simulink model "mytopologybat"  (R2014b)
settings: Solver=ode23tb  StartTime=0.0  StopTime=1  MaxStep=0.0001  MinStep=0.00001  RelTol=1e-3
libraries: powerlib x130, simulink x45, powerlib_meascontrol x2
(part 1 of 2)
settings Model: Creator=HOME  LastModifiedBy=SELVA
settings DataIOCC: SignalLoggingSaveFormat=ModelDataLogs
settings OptimizationCC: ExpressionDepthLimit=2147483647
settings DebuggingCC: UnderspecifiedInitializationDetection=Classic  MergeDetectMultiDrivingBlocksExec=none  FcnCallInpInsideContextMsg=UseLocalSettings  StateNameClashWarn=warning
settings GRTTargetCC: CombineOutputUpdateFcns=off  GRTInterface=on

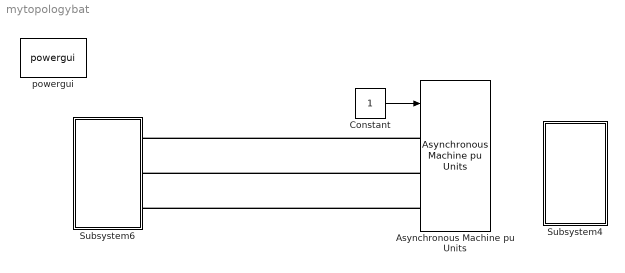
== system mytopologybat ==
  Asynchronous Machine pu Units : powerlib/Machines/Asynchronous Machine pu Units  PresetModel=No  MechanicalLoad=Torque Tm  ShowDetailedParameters=on  RotorType=Squirrel-cage  ReferenceFrame=Rotor  Units=pu  MeasurementBus=off  NominalParameters=[3730 460 60]  Stator=[0.01965 0.0397]  Rotor=[0.01909 0.0397]  Cage1=[0.01909 0.0397]  Cage2=[0.01909 0.0397]  Lm=1.354  Mechanical=[0.09526 0.05479 2]  PolePairs=2  InitialConditions="[ 1,0   0,0,0   0,0,0 ]"  SimulateSaturation=off  Saturation="[0.212,0.4201,0.8125,1.0979,1.4799,2.2457,3.2586,4.5763,6.4763 ;   0.5,0.7,0.9,1,1.1,1.2 ,1.3,1.4,1.5]"  LoadFlowParameters=0  TsPowergui=0  TsBlock=-1  IterativeModel=Trapezoidal non iterative  Pmec=0
  Constant : Constant
  Subsystem4 : Subsystem
  Subsystem6 : Subsystem  mask{m=1, fc=1000, v=230, c1=48}
      mask prompts: m "Modulation Index"; fc "Switching Frequency"; v "1 Phase Input Voltage"; c1 "DC Link Capacitor"
  powergui : powerlib/powergui  Priority=1  SimulationMode=Discrete  SolverType=Tustin/Backward Euler (TBE)  SampleTime=50e-6  frequency=60  SPID=off  DisableSnubberDevices=off  DisableRonSwitches=off  DisableVfSwitches=off  SwTol=0  DisplayEquations=off  Interpol=off  methode=off  Ts=100  frequencyindice=0  Pbase=100e6  ErrMax=1e-4  Iterations=50  UnitsV=kV  UnitsW=MW  FunctionMessages=off  echomessages=off  HookPort=off  EnableUseOfTLC=off  x0status=blocks  RestoreLinks=warning  ResistiveCurrentMeasurement=off  Frange=[0:2:500]  Ylog=off  Xlog=on  ShowGrid=off  save=off  variable=ZData  structure=ScopeData1  ZoomFFT=off  StartTime=0.1  cycles=1  DisplayStyle=1  fundamental=50  FreqAxis=off  MaxFrequency=1000  frequencyindicesteady=1  RmsSteady=1  display=off
  wires:
  Constant/1 -> Asynchronous Machine pu Units/1
  connections:
  Asynchronous Machine pu Units/LConn1 -- Subsystem6/RConn1
  Asynchronous Machine pu Units/LConn2 -- Subsystem6/RConn2
  Asynchronous Machine pu Units/LConn3 -- Subsystem6/RConn3

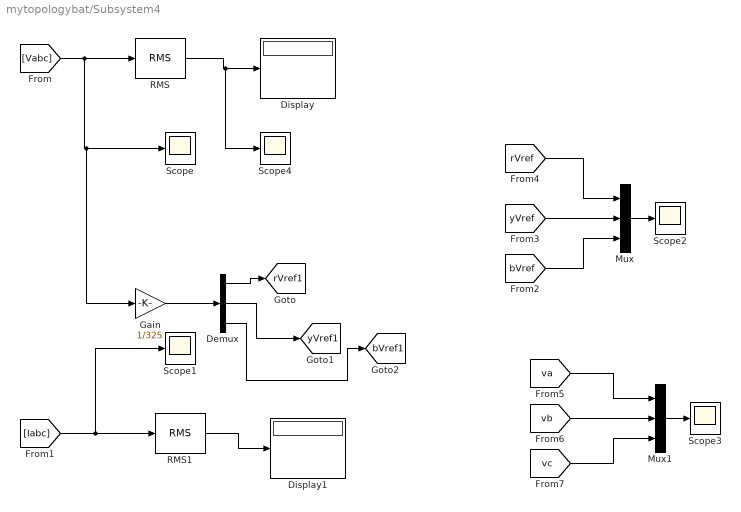
== system mytopologybat/Subsystem4 ==
  Demux : Demux  Outputs=3
  Display : Display
  Display1 : Display
  Gain : Gain  Gain=1/325
  Mux : Mux  Inputs=3
  Mux1 : Mux  Inputs=3
  RMS : powerlib_meascontrol/Measurements/RMS  TrueRMS=on  Freq=50  RMSInit=120  Ts=0
  RMS1 : powerlib_meascontrol/Measurements/RMS  TrueRMS=on  Freq=50  RMSInit=120  Ts=0
  Scope{,1..4} (5 alike) : Scope
      Scope settings: YMin=-400  YMax=400
      Scope1 settings: YMin=-600  YMax=800  SaveName=ScopeData2
      Scope2 settings: YMin=-8  YMax=8  SaveName=ScopeData4
      Scope3 settings: YMin=-400  YMax=400
      Scope4 settings: YMin=-600  YMax=600  SaveName=ScopeData3
  tag scope: bVref1=global, rVref1=global, yVref1=global
  wires:
  [Vabc] -> Gain/1, Scope/1, RMS/1
  RMS/1 -> Scope4/1, Display/1
  RMS1/1 -> Display1/1
  Mux/1 -> Scope2/1
  [bVref] -> Mux/3
  [rVref] -> Mux/1
  [yVref] -> Mux/2
  Mux1/1 -> Scope3/1
  [vc] -> Mux1/3
  [vb] -> Mux1/2
  [va] -> Mux1/1
  [Iabc] -> RMS1/1, Scope1/1
  Demux/1 -> [rVref1]
  Demux/2 -> [yVref1]
  Demux/3 -> [bVref1]
  Gain/1 -> Demux/1

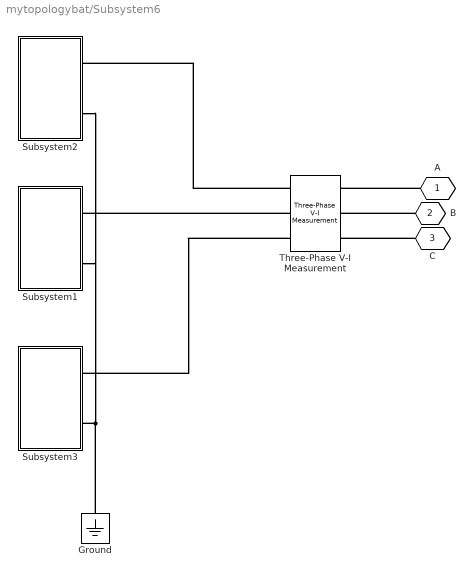
== system mytopologybat/Subsystem6 ==
  Ground : powerlib/Elements/Ground  LConnTagsString=a
  Subsystem1 : Subsystem
  Subsystem2 : Subsystem
  Subsystem3 : Subsystem
  Three-Phase V-I Measurement : powerlib/Measurements/Three-Phase V-I Measurement  VoltageMeasurement=phase-to-ground  SetLabelV=on  LabelV=Vabc  Vpu=off  VpuLL=off  CurrentMeasurement=yes  SetLabelI=on  LabelI=Iabc  Ipu=off  Pbase=100e6  Vbase=500e3  OutputType=Complex  PhasorSimulation=off  PSBequivalent=0
  A : PMIOPort  Port=1  Side=Right
  B : PMIOPort  Port=2  Side=Right
  C : PMIOPort  Port=3  Side=Right
  connections:
  Subsystem3/RConn2 -- Ground/LConn1 -- Subsystem2/RConn2 -- Subsystem1/RConn2
  Three-Phase V-I Measurement/LConn3 -- Subsystem3/RConn1
  Three-Phase V-I Measurement/LConn2 -- Subsystem1/RConn1
  Three-Phase V-I Measurement/LConn1 -- Subsystem2/RConn1
  A/RConn1 -- Three-Phase V-I Measurement/RConn1
  B/RConn1 -- Three-Phase V-I Measurement/RConn2
  C/RConn1 -- Three-Phase V-I Measurement/RConn3

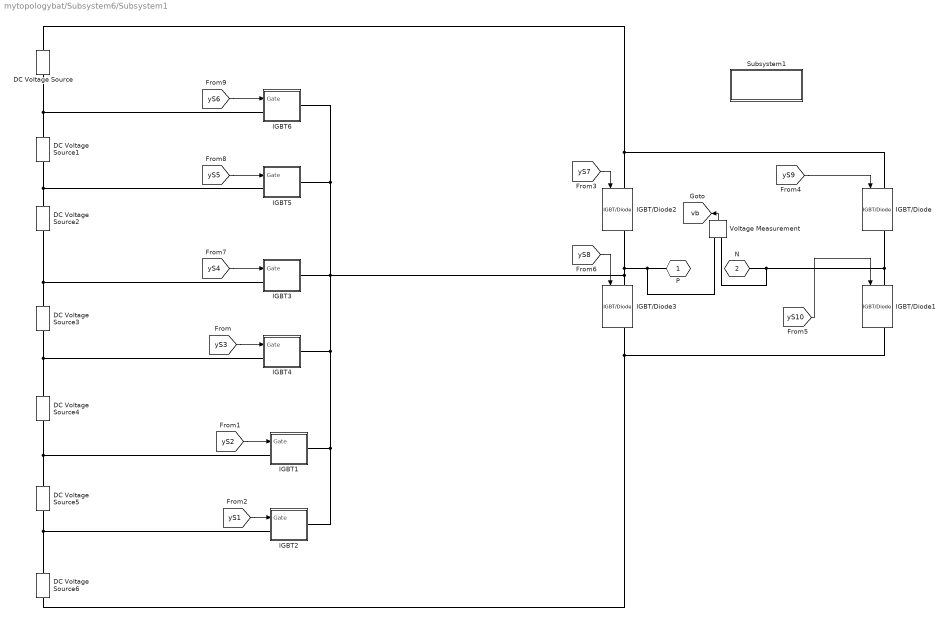
== system mytopologybat/Subsystem6/Subsystem1 ==
  DC Voltage Source{,1..6} (7 alike) : powerlib/Electrical Sources/DC Voltage Source  Amplitude=c1  Measurements=None
  IGBT/Diode{,1..3} (4 alike) : powerlib/Power Electronics/IGBT//Diode  Ron=1e-3  Rs=1e5  Cs=inf  Measurements=on
  IGBT1 : Subsystem
  IGBT2 : Subsystem
  IGBT3 : Subsystem
  IGBT4 : Subsystem
  IGBT5 : Subsystem
  IGBT6 : Subsystem
  Subsystem1 : Subsystem
  Voltage Measurement : powerlib/Measurements/Voltage Measurement  PhasorSimulation=off  OutputType=Complex  PSBequivalent=0
  P : PMIOPort  Port=1  Side=Right
  N : PMIOPort  Port=2  Side=Right
  tag scope: vb=global
  wires:
  [yS8] -> IGBT/Diode3/1
  [yS7] -> IGBT/Diode2/1
  [yS10] -> IGBT/Diode1/1
  [yS9] -> IGBT/Diode/1
  [yS1] -> IGBT2/1(Gate)
  [yS3] -> IGBT4/1(Gate)
  [yS2] -> IGBT1/1(Gate)
  [yS4] -> IGBT3/1(Gate)
  [yS5] -> IGBT5/1(Gate)
  [yS6] -> IGBT6/1(Gate)
  Voltage Measurement/1 -> [vb]
  connections:
  N/RConn1 -- IGBT/Diode/RConn1 -- IGBT/Diode1/LConn1 -- Voltage Measurement/LConn2
  IGBT/Diode3/RConn1 -- IGBT/Diode1/RConn1 -- DC Voltage Source6/LConn1
  IGBT2/RConn1 -- IGBT/Diode3/LConn1 -- Voltage Measurement/LConn1 -- P/RConn1 -- IGBT/Diode2/RConn1 -- IGBT6/RConn1 -- IGBT5/RConn1 -- IGBT3/RConn1 -- IGBT4/RConn1 -- IGBT1/RConn1
  IGBT/Diode2/LConn1 -- DC Voltage Source/RConn1 -- IGBT/Diode/LConn1
  DC Voltage Source4/RConn1 -- DC Voltage Source3/LConn1 -- IGBT4/LConn1
  DC Voltage Source5/RConn1 -- IGBT1/LConn1 -- DC Voltage Source4/LConn1
  DC Voltage Source5/LConn1 -- IGBT2/LConn1 -- DC Voltage Source6/RConn1
  DC Voltage Source/LConn1 -- IGBT6/LConn1 -- DC Voltage Source1/RConn1
  DC Voltage Source3/RConn1 -- DC Voltage Source2/LConn1 -- IGBT3/LConn1
  DC Voltage Source2/RConn1 -- DC Voltage Source1/LConn1 -- IGBT5/LConn1

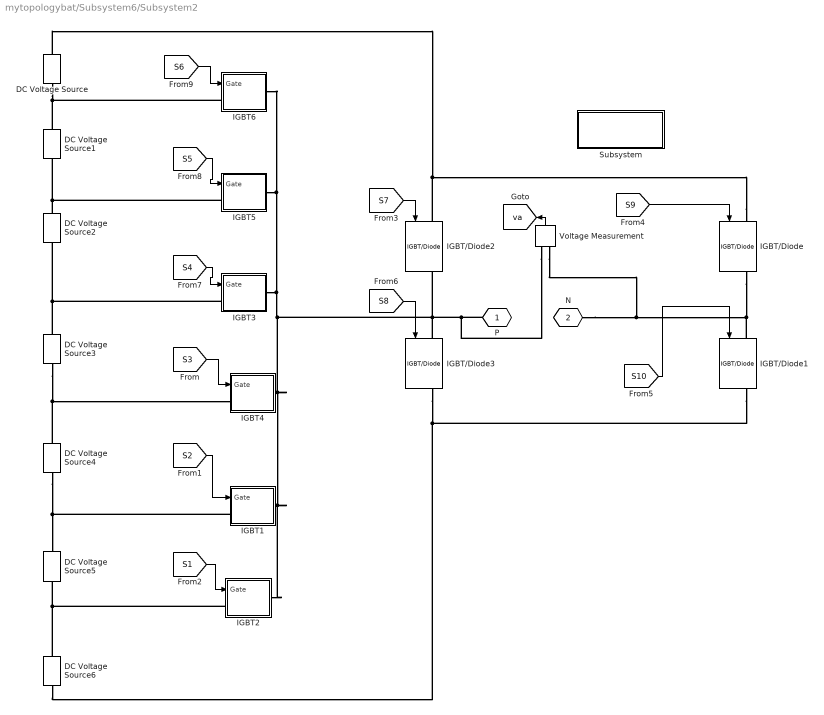
== system mytopologybat/Subsystem6/Subsystem2 ==
  DC Voltage Source{,1..6} (7 alike) : powerlib/Electrical Sources/DC Voltage Source  Amplitude=c1  Measurements=None
  IGBT/Diode{,1..3} (4 alike) : powerlib/Power Electronics/IGBT//Diode  Ron=1e-3  Rs=1e5  Cs=inf  Measurements=on
  IGBT1 : Subsystem
  IGBT2 : Subsystem
  IGBT3 : Subsystem
  IGBT4 : Subsystem
  IGBT5 : Subsystem
  IGBT6 : Subsystem
  Subsystem : Subsystem
  Voltage Measurement : powerlib/Measurements/Voltage Measurement  PhasorSimulation=off  OutputType=Complex  PSBequivalent=0
  P : PMIOPort  Port=1  Side=Right
  N : PMIOPort  Port=2  Side=Right
  tag scope: va=global
  wires:
  [S2] -> IGBT1/1(Gate)
  [S3] -> IGBT4/1(Gate)
  [S1] -> IGBT2/1(Gate)
  [S9] -> IGBT/Diode/1
  [S10] -> IGBT/Diode1/1
  [S7] -> IGBT/Diode2/1
  [S8] -> IGBT/Diode3/1
  [S4] -> IGBT3/1(Gate)
  [S5] -> IGBT5/1(Gate)
  [S6] -> IGBT6/1(Gate)
  Voltage Measurement/1 -> [va]
  connections:
  DC Voltage Source4/RConn1 -- DC Voltage Source3/LConn1 -- IGBT4/LConn1
  IGBT1/LConn1 -- DC Voltage Source4/LConn1 -- DC Voltage Source5/RConn1
  IGBT/Diode/LConn1 -- DC Voltage Source/RConn1 -- IGBT/Diode2/LConn1
  IGBT/Diode3/LConn1 -- Voltage Measurement/LConn1 -- P/RConn1 -- IGBT4/RConn1 -- IGBT2/RConn1 -- IGBT1/RConn1 -- IGBT6/RConn1 -- IGBT5/RConn1 -- IGBT3/RConn1 -- IGBT/Diode2/RConn1
  IGBT2/LConn1 -- DC Voltage Source6/RConn1 -- DC Voltage Source5/LConn1
  IGBT/Diode1/RConn1 -- DC Voltage Source6/LConn1 -- IGBT/Diode3/RConn1
  IGBT/Diode/RConn1 -- Voltage Measurement/LConn2 -- N/RConn1 -- IGBT/Diode1/LConn1
  IGBT6/LConn1 -- DC Voltage Source1/RConn1 -- DC Voltage Source/LConn1
  IGBT3/LConn1 -- DC Voltage Source3/RConn1 -- DC Voltage Source2/LConn1
  DC Voltage Source2/RConn1 -- DC Voltage Source1/LConn1 -- IGBT5/LConn1

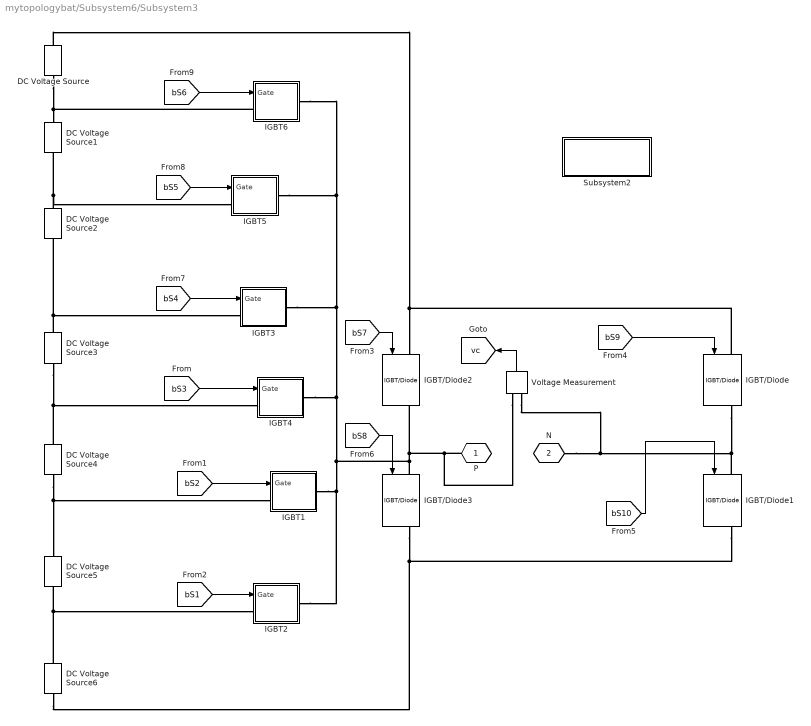
== system mytopologybat/Subsystem6/Subsystem3 ==
  DC Voltage Source{,1..6} (7 alike) : powerlib/Electrical Sources/DC Voltage Source  Amplitude=c1  Measurements=None
  IGBT/Diode{,1..3} (4 alike) : powerlib/Power Electronics/IGBT//Diode  Ron=1e-3  Rs=1e5  Cs=inf  Measurements=on
  IGBT1 : Subsystem
  IGBT2 : Subsystem
  IGBT3 : Subsystem
  IGBT4 : Subsystem
  IGBT5 : Subsystem
  IGBT6 : Subsystem
  Subsystem2 : Subsystem
  Voltage Measurement : powerlib/Measurements/Voltage Measurement  PhasorSimulation=off  OutputType=Complex  PSBequivalent=0
  P : PMIOPort  Port=1  Side=Right
  N : PMIOPort  Port=2  Side=Right
  tag scope: vc=global
  wires:
  [bS2] -> IGBT1/1(Gate)
  [bS3] -> IGBT4/1(Gate)
  [bS1] -> IGBT2/1(Gate)
  [bS9] -> IGBT/Diode/1
  [bS10] -> IGBT/Diode1/1
  [bS7] -> IGBT/Diode2/1
  [bS8] -> IGBT/Diode3/1
  [bS4] -> IGBT3/1(Gate)
  [bS5] -> IGBT5/1(Gate)
  [bS6] -> IGBT6/1(Gate)
  Voltage Measurement/1 -> [vc]
  connections:
  IGBT/Diode/LConn1 -- DC Voltage Source/RConn1 -- IGBT/Diode2/LConn1
  P/RConn1 -- Voltage Measurement/LConn1 -- IGBT/Diode2/RConn1 -- IGBT/Diode3/LConn1 -- IGBT6/RConn1 -- IGBT5/RConn1 -- IGBT3/RConn1 -- IGBT4/RConn1 -- IGBT1/RConn1 -- IGBT2/RConn1
  IGBT/Diode3/RConn1 -- DC Voltage Source6/LConn1 -- IGBT/Diode1/RConn1
  IGBT/Diode1/LConn1 -- Voltage Measurement/LConn2 -- N/RConn1 -- IGBT/Diode/RConn1
  DC Voltage Source4/RConn1 -- DC Voltage Source3/LConn1 -- IGBT4/LConn1
  DC Voltage Source4/LConn1 -- DC Voltage Source5/RConn1 -- IGBT1/LConn1
  DC Voltage Source5/LConn1 -- IGBT2/LConn1 -- DC Voltage Source6/RConn1
  DC Voltage Source/LConn1 -- IGBT6/LConn1 -- DC Voltage Source1/RConn1
  DC Voltage Source3/RConn1 -- DC Voltage Source2/LConn1 -- IGBT3/LConn1
  DC Voltage Source2/RConn1 -- IGBT5/LConn1 -- DC Voltage Source1/LConn1

== system mytopologybat/Subsystem6/Subsystem1/IGBT1 ==
  Gate : Inport
  Diode{,1..3} (4 alike) : powerlib/Power Electronics/Diode  Ron=0.001  Lon=0  Vf=0.8  IC=0  UseSnubber=off  Rs=500  Cs=250e-9  Measurements=on
  IGBT/Diode : powerlib/Power Electronics/IGBT//Diode  Ron=1e-3  Rs=1e5  Cs=inf  Measurements=on
  C : PMIOPort  Port=1  Side=Left
  E : PMIOPort  Port=2  Side=Right
  wires:
  Gate/1 -> IGBT/Diode/1
  connections:
  Diode/RConn1 -- Diode2/RConn1 -- IGBT/Diode/LConn1
  Diode1/LConn1 -- Diode3/LConn1 -- IGBT/Diode/RConn1
  Diode2/LConn1 -- Diode3/RConn1 -- C/RConn1
  Diode1/RConn1 -- Diode/LConn1 -- E/RConn1

== system mytopologybat/Subsystem6/Subsystem1/IGBT2 ==
  Gate : Inport
  Diode{,1..3} (4 alike) : powerlib/Power Electronics/Diode  Ron=0.001  Lon=0  Vf=0.8  IC=0  UseSnubber=off  Rs=500  Cs=250e-9  Measurements=on
  IGBT/Diode : powerlib/Power Electronics/IGBT//Diode  Ron=1e-3  Rs=1e5  Cs=inf  Measurements=on
  C : PMIOPort  Port=1  Side=Left
  E : PMIOPort  Port=2  Side=Right
  wires:
  Gate/1 -> IGBT/Diode/1
  connections:
  E/RConn1 -- Diode/LConn1 -- Diode1/RConn1
  C/RConn1 -- Diode3/RConn1 -- Diode2/LConn1
  IGBT/Diode/RConn1 -- Diode3/LConn1 -- Diode1/LConn1
  IGBT/Diode/LConn1 -- Diode2/RConn1 -- Diode/RConn1

== system mytopologybat/Subsystem6/Subsystem1/IGBT3 ==
  Gate : Inport
  Diode{,1..3} (4 alike) : powerlib/Power Electronics/Diode  Ron=0.001  Lon=0  Vf=0.8  IC=0  UseSnubber=off  Rs=500  Cs=250e-9  Measurements=on
  IGBT/Diode : powerlib/Power Electronics/IGBT//Diode  Ron=1e-3  Rs=1e5  Cs=inf  Measurements=on
  C : PMIOPort  Port=1  Side=Left
  E : PMIOPort  Port=2  Side=Right
  wires:
  Gate/1 -> IGBT/Diode/1
  connections:
  Diode/RConn1 -- Diode2/RConn1 -- IGBT/Diode/LConn1
  Diode1/LConn1 -- Diode3/LConn1 -- IGBT/Diode/RConn1
  Diode2/LConn1 -- Diode3/RConn1 -- C/RConn1
  Diode1/RConn1 -- Diode/LConn1 -- E/RConn1

== system mytopologybat/Subsystem6/Subsystem1/IGBT4 ==
  Gate : Inport
  Diode{,1..3} (4 alike) : powerlib/Power Electronics/Diode  Ron=0.001  Lon=0  Vf=0.8  IC=0  UseSnubber=off  Rs=500  Cs=250e-9  Measurements=on
  IGBT/Diode : powerlib/Power Electronics/IGBT//Diode  Ron=1e-3  Rs=1e5  Cs=inf  Measurements=on
  C : PMIOPort  Port=1  Side=Left
  E : PMIOPort  Port=2  Side=Right
  wires:
  Gate/1 -> IGBT/Diode/1
  connections:
  E/RConn1 -- Diode/LConn1 -- Diode1/RConn1
  C/RConn1 -- Diode3/RConn1 -- Diode2/LConn1
  IGBT/Diode/RConn1 -- Diode3/LConn1 -- Diode1/LConn1
  IGBT/Diode/LConn1 -- Diode2/RConn1 -- Diode/RConn1

== system mytopologybat/Subsystem6/Subsystem1/IGBT5 ==
  Gate : Inport
  Diode{,1..3} (4 alike) : powerlib/Power Electronics/Diode  Ron=0.001  Lon=0  Vf=0.8  IC=0  UseSnubber=off  Rs=500  Cs=250e-9  Measurements=on
  IGBT/Diode : powerlib/Power Electronics/IGBT//Diode  Ron=1e-3  Rs=1e5  Cs=inf  Measurements=on
  C : PMIOPort  Port=1  Side=Left
  E : PMIOPort  Port=2  Side=Right
  wires:
  Gate/1 -> IGBT/Diode/1
  connections:
  E/RConn1 -- Diode/LConn1 -- Diode1/RConn1
  C/RConn1 -- Diode3/RConn1 -- Diode2/LConn1
  IGBT/Diode/RConn1 -- Diode3/LConn1 -- Diode1/LConn1
  IGBT/Diode/LConn1 -- Diode2/RConn1 -- Diode/RConn1

== system mytopologybat/Subsystem6/Subsystem1/IGBT6 ==
  Gate : Inport
  Diode{,1..3} (4 alike) : powerlib/Power Electronics/Diode  Ron=0.001  Lon=0  Vf=0.8  IC=0  UseSnubber=off  Rs=500  Cs=250e-9  Measurements=on
  IGBT/Diode : powerlib/Power Electronics/IGBT//Diode  Ron=1e-3  Rs=1e5  Cs=inf  Measurements=on
  C : PMIOPort  Port=1  Side=Left
  E : PMIOPort  Port=2  Side=Right
  wires:
  Gate/1 -> IGBT/Diode/1
  connections:
  Diode/RConn1 -- Diode2/RConn1 -- IGBT/Diode/LConn1
  Diode1/LConn1 -- Diode3/LConn1 -- IGBT/Diode/RConn1
  Diode2/LConn1 -- Diode3/RConn1 -- C/RConn1
  Diode1/RConn1 -- Diode/LConn1 -- E/RConn1

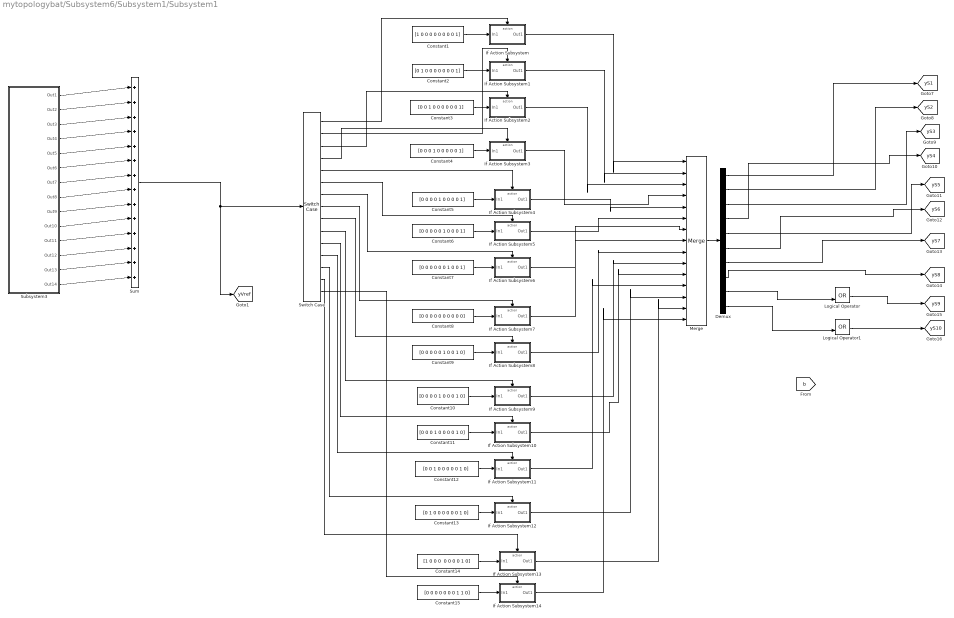
== system mytopologybat/Subsystem6/Subsystem1/Subsystem1 ==
  Constant1 : Constant  Value=[1 0 0 0 0 0 0 0 0 1]
  Constant10 : Constant  Value=[0 0 0 0 1 0 0 0 1 0]
  Constant11 : Constant  Value=[0 0 0 1 0 0 0 0 1 0]
  Constant12 : Constant  Value=[0 0 1 0 0 0 0 0 1 0]
  Constant13 : Constant  Value=[0 1 0 0 0 0 0 0 1 0]
  Constant14 : Constant  Value="[1 0 0 0  0 0 0 0 1 0]"
  Constant15 : Constant  Value=[0 0 0 0 0 0 0 1 1 0]
  Constant2 : Constant  Value=[0 1 0 0 0 0 0 0 0 1]
  Constant3 : Constant  Value=[0 0 1 0 0 0 0 0 0 1]
  Constant4 : Constant  Value=[0 0 0 1 0 0 0 0 0 1]
  Constant5 : Constant  Value=[0 0 0 0 1 0 0 0 0 1]
  Constant6 : Constant  Value=[0 0 0 0 0 1 0 0 0 1]
  Constant7 : Constant  Value=[0 0 0 0 0 0 1 0 0 1]
  Constant8 : Constant  Value=[0 0 0 0 0 0 0 0 0 0]
  Constant9 : Constant  Value=[0 0 0 0 0 1 0 0 1 0]
  Demux : Demux  Outputs=10
  If Action Subsystem : Subsystem  TreatAsAtomicUnit=on
  If Action Subsystem1 : Subsystem  TreatAsAtomicUnit=on
  If Action Subsystem10 : Subsystem  TreatAsAtomicUnit=on
  If Action Subsystem11 : Subsystem  TreatAsAtomicUnit=on
  If Action Subsystem12 : Subsystem  TreatAsAtomicUnit=on
  If Action Subsystem13 : Subsystem  TreatAsAtomicUnit=on
  If Action Subsystem14 : Subsystem  TreatAsAtomicUnit=on
  If Action Subsystem2 : Subsystem  TreatAsAtomicUnit=on
  If Action Subsystem3 : Subsystem  TreatAsAtomicUnit=on
  If Action Subsystem4 : Subsystem  TreatAsAtomicUnit=on
  If Action Subsystem5 : Subsystem  TreatAsAtomicUnit=on
  If Action Subsystem6 : Subsystem  TreatAsAtomicUnit=on
  If Action Subsystem7 : Subsystem  TreatAsAtomicUnit=on
  If Action Subsystem8 : Subsystem  TreatAsAtomicUnit=on
  If Action Subsystem9 : Subsystem  TreatAsAtomicUnit=on
  Logical Operator : Logic  Operator=OR  AllPortsSameDT=off  OutDataTypeStr=boolean
  Logical Operator1 : Logic  Operator=OR  AllPortsSameDT=off  OutDataTypeStr=boolean
  Merge : Merge  Inputs=15
  Subsystem3 : Subsystem
  Sum : Sum  Inputs=|++++++++++++++
  Switch Case : SwitchCase  CaseConditions={1 2 3 4 5 6 7 0 -1 -2 -3 -4 -5 -6 -7}  ShowDefaultCase=off
  tag scope: yS10=global, yS1=global, yS2=global, yS3=global, yS4=global, yS5=global, yS6=global, yS7=global, yS8=global, yS9=global, yVref=global
  wires:
  Constant1/1 -> If Action Subsystem/1(In1)
  Constant2/1 -> If Action Subsystem1/1(In1)
  Constant3/1 -> If Action Subsystem2/1(In1)
  Constant4/1 -> If Action Subsystem3/1(In1)
  Constant5/1 -> If Action Subsystem4/1(In1)
  If Action Subsystem/1(Out1) -> Merge/1
  If Action Subsystem1/1(Out1) -> Merge/2
  If Action Subsystem2/1(Out1) -> Merge/3
  If Action Subsystem3/1(Out1) -> Merge/4
  If Action Subsystem4/1(Out1) -> Merge/5
  Merge/1 -> Demux/1
  Demux/3 -> [yS3]
  Demux/4 -> [yS4]
  Demux/1 -> [yS1]
  Demux/5 -> [yS5]
  Constant6/1 -> If Action Subsystem5/1(In1)
  Constant7/1 -> If Action Subsystem6/1(In1)
  If Action Subsystem6/1(Out1) -> Merge/7
  If Action Subsystem5/1(Out1) -> Merge/6
  Demux/6 -> [yS6]
  Demux/7 -> [yS7]
  Constant8/1 -> If Action Subsystem7/1(In1)
  Constant9/1 -> If Action Subsystem8/1(In1)
  If Action Subsystem8/1(Out1) -> Merge/9
  If Action Subsystem7/1(Out1) -> Merge/8
  Sum/1 -> [yVref], Switch Case/1
  Switch Case/1 -> If Action Subsystem/Action
  Switch Case/2 -> If Action Subsystem1/Action
  Switch Case/3 -> If Action Subsystem2/Action
  Switch Case/4 -> If Action Subsystem3/Action
  Switch Case/5 -> If Action Subsystem4/Action
  Switch Case/6 -> If Action Subsystem5/Action
  Switch Case/7 -> If Action Subsystem6/Action
  Switch Case/8 -> If Action Subsystem7/Action
  Switch Case/9 -> If Action Subsystem8/Action
  Constant10/1 -> If Action Subsystem9/1(In1)
  Constant11/1 -> If Action Subsystem10/1(In1)
  Constant12/1 -> If Action Subsystem11/1(In1)
  Constant13/1 -> If Action Subsystem12/1(In1)
  Constant14/1 -> If Action Subsystem13/1(In1)
  If Action Subsystem9/1(Out1) -> Merge/10
  If Action Subsystem10/1(Out1) -> Merge/11
  If Action Subsystem12/1(Out1) -> Merge/13
  If Action Subsystem13/1(Out1) -> Merge/14
  Constant15/1 -> If Action Subsystem14/1(In1)
  Switch Case/11 -> If Action Subsystem10/Action
  Switch Case/12 -> If Action Subsystem11/Action
  Switch Case/13 -> If Action Subsystem12/Action
  Switch Case/14 -> If Action Subsystem13/Action
  Switch Case/15 -> If Action Subsystem14/Action
  Switch Case/10 -> If Action Subsystem9/Action
  If Action Subsystem11/1(Out1) -> Merge/12
  If Action Subsystem14/1(Out1) -> Merge/15
  Demux/8 -> [yS8]
  Demux/2 -> [yS2]
  Subsystem3/1(Out1) -> Sum/1
  Subsystem3/6(Out6) -> Sum/6
  Subsystem3/7(Out7) -> Sum/7
  Subsystem3/10(Out10) -> Sum/10
  Subsystem3/9(Out9) -> Sum/9
  Subsystem3/8(Out8) -> Sum/8
  Subsystem3/5(Out5) -> Sum/5
  Subsystem3/4(Out4) -> Sum/4
  Subsystem3/2(Out2) -> Sum/2
  Subsystem3/3(Out3) -> Sum/3
  Subsystem3/14(Out14) -> Sum/14
  Subsystem3/12(Out12) -> Sum/12
  Subsystem3/13(Out13) -> Sum/13
  Subsystem3/11(Out11) -> Sum/11
  Demux/9 -> Logical Operator/2
  Logical Operator/1 -> [yS9]
  Logical Operator1/1 -> [yS10]
  Demux/10 -> Logical Operator1/2

== system mytopologybat/Subsystem6/Subsystem2/IGBT1 ==
  Gate : Inport
  Diode{,1..3} (4 alike) : powerlib/Power Electronics/Diode  Ron=0.001  Lon=0  Vf=0.8  IC=0  UseSnubber=off  Rs=500  Cs=250e-9  Measurements=on
  IGBT/Diode : powerlib/Power Electronics/IGBT//Diode  Ron=1e-3  Rs=1e5  Cs=inf  Measurements=on
  C : PMIOPort  Port=1  Side=Left
  E : PMIOPort  Port=2  Side=Right
  wires:
  Gate/1 -> IGBT/Diode/1
  connections:
  E/RConn1 -- Diode/LConn1 -- Diode1/RConn1
  C/RConn1 -- Diode3/RConn1 -- Diode2/LConn1
  IGBT/Diode/RConn1 -- Diode3/LConn1 -- Diode1/LConn1
  IGBT/Diode/LConn1 -- Diode2/RConn1 -- Diode/RConn1

== system mytopologybat/Subsystem6/Subsystem2/IGBT2 ==
  Gate : Inport
  Diode{,1..3} (4 alike) : powerlib/Power Electronics/Diode  Ron=0.001  Lon=0  Vf=0.8  IC=0  UseSnubber=off  Rs=500  Cs=250e-9  Measurements=on
  IGBT/Diode : powerlib/Power Electronics/IGBT//Diode  Ron=1e-3  Rs=1e5  Cs=inf  Measurements=on
  C : PMIOPort  Port=1  Side=Left
  E : PMIOPort  Port=2  Side=Right
  wires:
  Gate/1 -> IGBT/Diode/1
  connections:
  Diode/RConn1 -- Diode2/RConn1 -- IGBT/Diode/LConn1
  Diode1/LConn1 -- Diode3/LConn1 -- IGBT/Diode/RConn1
  Diode2/LConn1 -- Diode3/RConn1 -- C/RConn1
  Diode1/RConn1 -- Diode/LConn1 -- E/RConn1

== system mytopologybat/Subsystem6/Subsystem2/IGBT3 ==
  Gate : Inport
  Diode{,1..3} (4 alike) : powerlib/Power Electronics/Diode  Ron=0.001  Lon=0  Vf=0.8  IC=0  UseSnubber=off  Rs=500  Cs=250e-9  Measurements=on
  IGBT/Diode : powerlib/Power Electronics/IGBT//Diode  Ron=1e-3  Rs=1e5  Cs=inf  Measurements=on
  C : PMIOPort  Port=1  Side=Left
  E : PMIOPort  Port=2  Side=Right
  wires:
  Gate/1 -> IGBT/Diode/1
  connections:
  E/RConn1 -- Diode/LConn1 -- Diode1/RConn1
  C/RConn1 -- Diode3/RConn1 -- Diode2/LConn1
  IGBT/Diode/RConn1 -- Diode3/LConn1 -- Diode1/LConn1
  IGBT/Diode/LConn1 -- Diode2/RConn1 -- Diode/RConn1

== system mytopologybat/Subsystem6/Subsystem2/IGBT4 ==
  Gate : Inport
  Diode{,1..3} (4 alike) : powerlib/Power Electronics/Diode  Ron=0.001  Lon=0  Vf=0.8  IC=0  UseSnubber=off  Rs=500  Cs=250e-9  Measurements=on
  IGBT/Diode : powerlib/Power Electronics/IGBT//Diode  Ron=1e-3  Rs=1e5  Cs=inf  Measurements=on
  C : PMIOPort  Port=1  Side=Left
  E : PMIOPort  Port=2  Side=Right
  wires:
  Gate/1 -> IGBT/Diode/1
  connections:
  Diode/RConn1 -- Diode2/RConn1 -- IGBT/Diode/LConn1
  Diode1/LConn1 -- Diode3/LConn1 -- IGBT/Diode/RConn1
  Diode2/LConn1 -- Diode3/RConn1 -- C/RConn1
  Diode1/RConn1 -- Diode/LConn1 -- E/RConn1

== system mytopologybat/Subsystem6/Subsystem2/IGBT5 ==
  Gate : Inport
  Diode{,1..3} (4 alike) : powerlib/Power Electronics/Diode  Ron=0.001  Lon=0  Vf=0.8  IC=0  UseSnubber=off  Rs=500  Cs=250e-9  Measurements=on
  IGBT/Diode : powerlib/Power Electronics/IGBT//Diode  Ron=1e-3  Rs=1e5  Cs=inf  Measurements=on
  C : PMIOPort  Port=1  Side=Left
  E : PMIOPort  Port=2  Side=Right
  wires:
  Gate/1 -> IGBT/Diode/1
  connections:
  Diode/RConn1 -- Diode2/RConn1 -- IGBT/Diode/LConn1
  Diode1/LConn1 -- Diode3/LConn1 -- IGBT/Diode/RConn1
  Diode2/LConn1 -- Diode3/RConn1 -- C/RConn1
  Diode1/RConn1 -- Diode/LConn1 -- E/RConn1

== system mytopologybat/Subsystem6/Subsystem2/IGBT6 ==
  Gate : Inport
  Diode{,1..3} (4 alike) : powerlib/Power Electronics/Diode  Ron=0.001  Lon=0  Vf=0.8  IC=0  UseSnubber=off  Rs=500  Cs=250e-9  Measurements=on
  IGBT/Diode : powerlib/Power Electronics/IGBT//Diode  Ron=1e-3  Rs=1e5  Cs=inf  Measurements=on
  C : PMIOPort  Port=1  Side=Left
  E : PMIOPort  Port=2  Side=Right
  wires:
  Gate/1 -> IGBT/Diode/1
  connections:
  E/RConn1 -- Diode/LConn1 -- Diode1/RConn1
  C/RConn1 -- Diode3/RConn1 -- Diode2/LConn1
  IGBT/Diode/RConn1 -- Diode3/LConn1 -- Diode1/LConn1
  IGBT/Diode/LConn1 -- Diode2/RConn1 -- Diode/RConn1

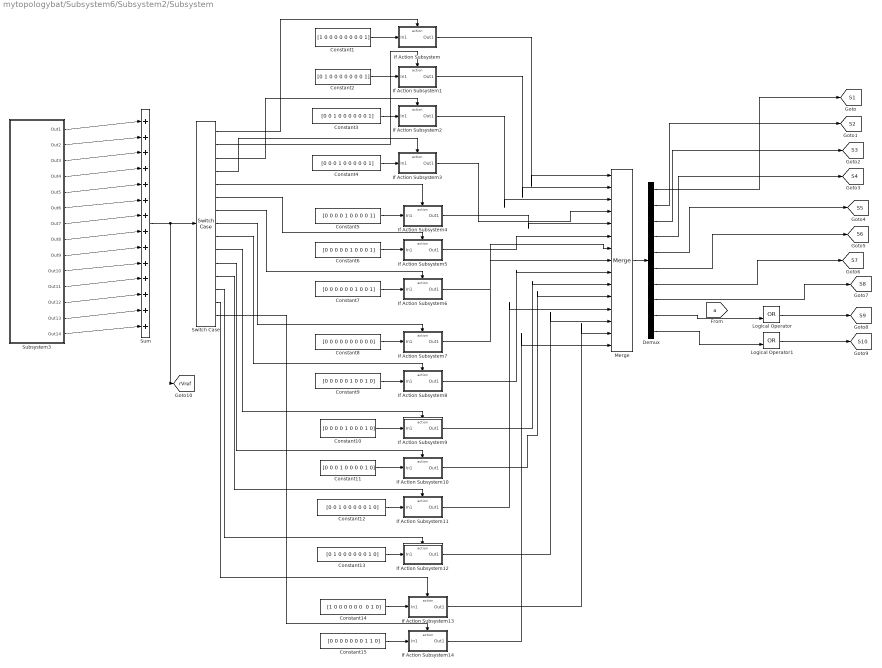
== system mytopologybat/Subsystem6/Subsystem2/Subsystem ==
  Constant1 : Constant  Value=[1 0 0 0 0 0 0 0 0 1]
  Constant10 : Constant  Value=[0 0 0 0 1 0 0 0 1 0]
  Constant11 : Constant  Value=[0 0 0 1 0 0 0 0 1 0]
  Constant12 : Constant  Value=[0 0 1 0 0 0 0 0 1 0]
  Constant13 : Constant  Value=[0 1 0 0 0 0 0 0 1 0]
  Constant14 : Constant  Value="[1 0 0 0 0 0 0  0 1 0]"
  Constant15 : Constant  Value=[0 0 0 0 0 0 0 1 1 0]
  Constant2 : Constant  Value=[0 1 0 0 0 0 0 0 0 1]
  Constant3 : Constant  Value=[0 0 1 0 0 0 0 0 0 1]
  Constant4 : Constant  Value=[0 0 0 1 0 0 0 0 0 1]
  Constant5 : Constant  Value=[0 0 0 0 1 0 0 0 0 1]
  Constant6 : Constant  Value=[0 0 0 0 0 1 0 0 0 1]
  Constant7 : Constant  Value=[0 0 0 0 0 0 1 0 0 1]
  Constant8 : Constant  Value=[0 0 0 0 0 0 0 0 0 0]
  Constant9 : Constant  Value=[0 0 0 0 0 1 0 0 1 0]
  Demux : Demux  Outputs=10
  If Action Subsystem : Subsystem  TreatAsAtomicUnit=on
  If Action Subsystem1 : Subsystem  TreatAsAtomicUnit=on
  If Action Subsystem10 : Subsystem  TreatAsAtomicUnit=on
  If Action Subsystem11 : Subsystem  TreatAsAtomicUnit=on
  If Action Subsystem12 : Subsystem  TreatAsAtomicUnit=on
  If Action Subsystem13 : Subsystem  TreatAsAtomicUnit=on
  If Action Subsystem14 : Subsystem  TreatAsAtomicUnit=on
  If Action Subsystem2 : Subsystem  TreatAsAtomicUnit=on
  If Action Subsystem3 : Subsystem  TreatAsAtomicUnit=on
  If Action Subsystem4 : Subsystem  TreatAsAtomicUnit=on
  If Action Subsystem5 : Subsystem  TreatAsAtomicUnit=on
  If Action Subsystem6 : Subsystem  TreatAsAtomicUnit=on
  If Action Subsystem7 : Subsystem  TreatAsAtomicUnit=on
  If Action Subsystem8 : Subsystem  TreatAsAtomicUnit=on
  If Action Subsystem9 : Subsystem  TreatAsAtomicUnit=on
  Logical Operator : Logic  Operator=OR  AllPortsSameDT=off  OutDataTypeStr=boolean
  Logical Operator1 : Logic  Operator=OR  AllPortsSameDT=off  OutDataTypeStr=boolean
  Merge : Merge  Inputs=15
  Subsystem3 : Subsystem
  Sum : Sum  Inputs=|++++++++++++++
  Switch Case : SwitchCase  CaseConditions={1 2 3 4 5 6 7 0 -1 -2 -3 -4 -5 -6 -7}  ShowDefaultCase=off
  tag scope: S10=global, S1=global, S2=global, S3=global, S4=global, S5=global, S6=global, S7=global, S8=global, S9=global, rVref=global
  wires:
  Constant1/1 -> If Action Subsystem/1(In1)
  Constant2/1 -> If Action Subsystem1/1(In1)
  Constant3/1 -> If Action Subsystem2/1(In1)
  Constant4/1 -> If Action Subsystem3/1(In1)
  Constant5/1 -> If Action Subsystem4/1(In1)
  If Action Subsystem/1(Out1) -> Merge/1
  If Action Subsystem1/1(Out1) -> Merge/2
  If Action Subsystem2/1(Out1) -> Merge/3
  If Action Subsystem3/1(Out1) -> Merge/4
  If Action Subsystem4/1(Out1) -> Merge/5
  Merge/1 -> Demux/1
  Demux/2 -> [S2]
  Demux/3 -> [S3]
  Demux/4 -> [S4]
  Demux/1 -> [S1]
  Demux/5 -> [S5]
  Constant6/1 -> If Action Subsystem5/1(In1)
  Constant7/1 -> If Action Subsystem6/1(In1)
  If Action Subsystem6/1(Out1) -> Merge/7
  If Action Subsystem5/1(Out1) -> Merge/6
  Demux/6 -> [S6]
  Demux/7 -> [S7]
  Constant8/1 -> If Action Subsystem7/1(In1)
  Constant9/1 -> If Action Subsystem8/1(In1)
  If Action Subsystem8/1(Out1) -> Merge/9
  If Action Subsystem7/1(Out1) -> Merge/8
  Switch Case/1 -> If Action Subsystem/Action
  Switch Case/2 -> If Action Subsystem1/Action
  Switch Case/3 -> If Action Subsystem2/Action
  Switch Case/4 -> If Action Subsystem3/Action
  Switch Case/5 -> If Action Subsystem4/Action
  Switch Case/6 -> If Action Subsystem5/Action
  Switch Case/7 -> If Action Subsystem6/Action
  Switch Case/8 -> If Action Subsystem7/Action
  Switch Case/9 -> If Action Subsystem8/Action
  Constant10/1 -> If Action Subsystem9/1(In1)
  Constant11/1 -> If Action Subsystem10/1(In1)
  Constant12/1 -> If Action Subsystem11/1(In1)
  Constant13/1 -> If Action Subsystem12/1(In1)
  Constant14/1 -> If Action Subsystem13/1(In1)
  If Action Subsystem9/1(Out1) -> Merge/10
  If Action Subsystem10/1(Out1) -> Merge/11
  If Action Subsystem12/1(Out1) -> Merge/13
  If Action Subsystem13/1(Out1) -> Merge/14
  Constant15/1 -> If Action Subsystem14/1(In1)
  Switch Case/11 -> If Action Subsystem10/Action
  Switch Case/12 -> If Action Subsystem11/Action
  Switch Case/13 -> If Action Subsystem12/Action
  Switch Case/14 -> If Action Subsystem13/Action
  Switch Case/15 -> If Action Subsystem14/Action
  Switch Case/10 -> If Action Subsystem9/Action
  If Action Subsystem11/1(Out1) -> Merge/12
  If Action Subsystem14/1(Out1) -> Merge/15
  Demux/8 -> [S8]
  Subsystem3/1(Out1) -> Sum/1
  Subsystem3/6(Out6) -> Sum/6
  Subsystem3/7(Out7) -> Sum/7
  Subsystem3/10(Out10) -> Sum/10
  Subsystem3/9(Out9) -> Sum/9
  Subsystem3/8(Out8) -> Sum/8
  Subsystem3/5(Out5) -> Sum/5
  Subsystem3/4(Out4) -> Sum/4
  Subsystem3/2(Out2) -> Sum/2
  Subsystem3/3(Out3) -> Sum/3
  Subsystem3/14(Out14) -> Sum/14
  Subsystem3/12(Out12) -> Sum/12
  Subsystem3/13(Out13) -> Sum/13
  Subsystem3/11(Out11) -> Sum/11
  Sum/1 -> [rVref], Switch Case/1
  Demux/9 -> Logical Operator/2
  Logical Operator/1 -> [S9]
  Logical Operator1/1 -> [S10]
  Demux/10 -> Logical Operator1/2

== system mytopologybat/Subsystem6/Subsystem3/IGBT1 ==
  Gate : Inport
  Diode{,1..3} (4 alike) : powerlib/Power Electronics/Diode  Ron=0.001  Lon=0  Vf=0.8  IC=0  UseSnubber=off  Rs=500  Cs=250e-9  Measurements=on
  IGBT/Diode : powerlib/Power Electronics/IGBT//Diode  Ron=1e-3  Rs=1e5  Cs=inf  Measurements=on
  C : PMIOPort  Port=1  Side=Left
  E : PMIOPort  Port=2  Side=Right
  wires:
  Gate/1 -> IGBT/Diode/1
  connections:
  E/RConn1 -- Diode/LConn1 -- Diode1/RConn1
  C/RConn1 -- Diode3/RConn1 -- Diode2/LConn1
  IGBT/Diode/RConn1 -- Diode3/LConn1 -- Diode1/LConn1
  IGBT/Diode/LConn1 -- Diode2/RConn1 -- Diode/RConn1

== system mytopologybat/Subsystem6/Subsystem3/IGBT2 ==
  Gate : Inport
  Diode{,1..3} (4 alike) : powerlib/Power Electronics/Diode  Ron=0.001  Lon=0  Vf=0.8  IC=0  UseSnubber=off  Rs=500  Cs=250e-9  Measurements=on
  IGBT/Diode : powerlib/Power Electronics/IGBT//Diode  Ron=1e-3  Rs=1e5  Cs=inf  Measurements=on
  C : PMIOPort  Port=1  Side=Left
  E : PMIOPort  Port=2  Side=Right
  wires:
  Gate/1 -> IGBT/Diode/1
  connections:
  Diode/RConn1 -- Diode2/RConn1 -- IGBT/Diode/LConn1
  Diode1/LConn1 -- Diode3/LConn1 -- IGBT/Diode/RConn1
  Diode2/LConn1 -- Diode3/RConn1 -- C/RConn1
  Diode1/RConn1 -- Diode/LConn1 -- E/RConn1

== system mytopologybat/Subsystem6/Subsystem3/IGBT3 ==
  Gate : Inport
  Diode{,1..3} (4 alike) : powerlib/Power Electronics/Diode  Ron=0.001  Lon=0  Vf=0.8  IC=0  UseSnubber=off  Rs=500  Cs=250e-9  Measurements=on
  IGBT/Diode : powerlib/Power Electronics/IGBT//Diode  Ron=1e-3  Rs=1e5  Cs=inf  Measurements=on
  C : PMIOPort  Port=1  Side=Left
  E : PMIOPort  Port=2  Side=Right
  wires:
  Gate/1 -> IGBT/Diode/1
  connections:
  E/RConn1 -- Diode/LConn1 -- Diode1/RConn1
  C/RConn1 -- Diode3/RConn1 -- Diode2/LConn1
  IGBT/Diode/RConn1 -- Diode3/LConn1 -- Diode1/LConn1
  IGBT/Diode/LConn1 -- Diode2/RConn1 -- Diode/RConn1

== system mytopologybat/Subsystem6/Subsystem3/IGBT4 ==
  Gate : Inport
  Diode{,1..3} (4 alike) : powerlib/Power Electronics/Diode  Ron=0.001  Lon=0  Vf=0.8  IC=0  UseSnubber=off  Rs=500  Cs=250e-9  Measurements=on
  IGBT/Diode : powerlib/Power Electronics/IGBT//Diode  Ron=1e-3  Rs=1e5  Cs=inf  Measurements=on
  C : PMIOPort  Port=1  Side=Left
  E : PMIOPort  Port=2  Side=Right
  wires:
  Gate/1 -> IGBT/Diode/1
  connections:
  Diode/RConn1 -- Diode2/RConn1 -- IGBT/Diode/LConn1
  Diode1/LConn1 -- Diode3/LConn1 -- IGBT/Diode/RConn1
  Diode2/LConn1 -- Diode3/RConn1 -- C/RConn1
  Diode1/RConn1 -- Diode/LConn1 -- E/RConn1

== system mytopologybat/Subsystem6/Subsystem3/IGBT5 ==
  Gate : Inport
  Diode{,1..3} (4 alike) : powerlib/Power Electronics/Diode  Ron=0.001  Lon=0  Vf=0.8  IC=0  UseSnubber=off  Rs=500  Cs=250e-9  Measurements=on
  IGBT/Diode : powerlib/Power Electronics/IGBT//Diode  Ron=1e-3  Rs=1e5  Cs=inf  Measurements=on
  C : PMIOPort  Port=1  Side=Left
  E : PMIOPort  Port=2  Side=Right
  wires:
  Gate/1 -> IGBT/Diode/1
  connections:
  Diode/RConn1 -- Diode2/RConn1 -- IGBT/Diode/LConn1
  Diode1/LConn1 -- Diode3/LConn1 -- IGBT/Diode/RConn1
  Diode2/LConn1 -- Diode3/RConn1 -- C/RConn1
  Diode1/RConn1 -- Diode/LConn1 -- E/RConn1

== system mytopologybat/Subsystem6/Subsystem3/IGBT6 ==
  Gate : Inport
  Diode{,1..3} (4 alike) : powerlib/Power Electronics/Diode  Ron=0.001  Lon=0  Vf=0.8  IC=0  UseSnubber=off  Rs=500  Cs=250e-9  Measurements=on
  IGBT/Diode : powerlib/Power Electronics/IGBT//Diode  Ron=1e-3  Rs=1e5  Cs=inf  Measurements=on
  C : PMIOPort  Port=1  Side=Left
  E : PMIOPort  Port=2  Side=Right
  wires:
  Gate/1 -> IGBT/Diode/1
  connections:
  E/RConn1 -- Diode/LConn1 -- Diode1/RConn1
  C/RConn1 -- Diode3/RConn1 -- Diode2/LConn1
  IGBT/Diode/RConn1 -- Diode3/LConn1 -- Diode1/LConn1
  IGBT/Diode/LConn1 -- Diode2/RConn1 -- Diode/RConn1

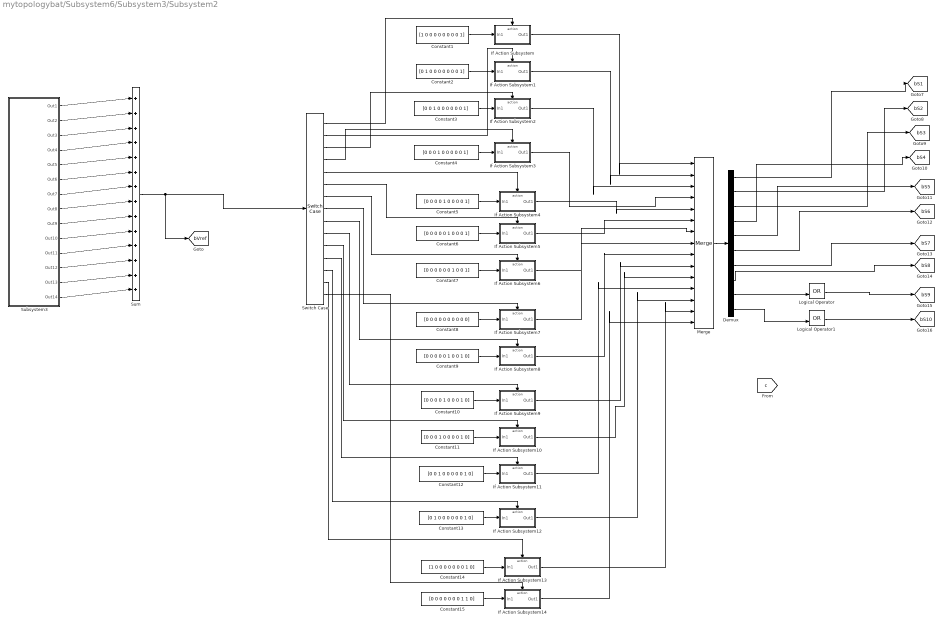
== system mytopologybat/Subsystem6/Subsystem3/Subsystem2 ==
  Constant1 : Constant  Value=[1 0 0 0 0 0 0 0 0 1]
  Constant10 : Constant  Value=[0 0 0 0 1 0 0 0 1 0]
  Constant11 : Constant  Value=[0 0 0 1 0 0 0 0 1 0]
  Constant12 : Constant  Value=[0 0 1 0 0 0 0 0 1 0]
  Constant13 : Constant  Value=[0 1 0 0 0 0 0 0 1 0]
  Constant14 : Constant  Value=[1 0 0 0 0 0 0 0 1 0]
  Constant15 : Constant  Value=[0 0 0 0 0 0 0 1 1 0]
  Constant2 : Constant  Value=[0 1 0 0 0 0 0 0 0 1]
  Constant3 : Constant  Value=[0 0 1 0 0 0 0 0 0 1]
  Constant4 : Constant  Value=[0 0 0 1 0 0 0 0 0 1]
  Constant5 : Constant  Value=[0 0 0 0 1 0 0 0 0 1]
  Constant6 : Constant  Value=[0 0 0 0 0 1 0 0 0 1]
  Constant7 : Constant  Value=[0 0 0 0 0 0 1 0 0 1]
  Constant8 : Constant  Value=[0 0 0 0 0 0 0 0 0 0]
  Constant9 : Constant  Value=[0 0 0 0 0 1 0 0 1 0]
  Demux : Demux  Outputs=10
  If Action Subsystem : Subsystem  TreatAsAtomicUnit=on
  If Action Subsystem1 : Subsystem  TreatAsAtomicUnit=on
  If Action Subsystem10 : Subsystem  TreatAsAtomicUnit=on
  If Action Subsystem11 : Subsystem  TreatAsAtomicUnit=on
  If Action Subsystem12 : Subsystem  TreatAsAtomicUnit=on
  If Action Subsystem13 : Subsystem  TreatAsAtomicUnit=on
  If Action Subsystem14 : Subsystem  TreatAsAtomicUnit=on
  If Action Subsystem2 : Subsystem  TreatAsAtomicUnit=on
  If Action Subsystem3 : Subsystem  TreatAsAtomicUnit=on
  If Action Subsystem4 : Subsystem  TreatAsAtomicUnit=on
  If Action Subsystem5 : Subsystem  TreatAsAtomicUnit=on
  If Action Subsystem6 : Subsystem  TreatAsAtomicUnit=on
  If Action Subsystem7 : Subsystem  TreatAsAtomicUnit=on
  If Action Subsystem8 : Subsystem  TreatAsAtomicUnit=on
  If Action Subsystem9 : Subsystem  TreatAsAtomicUnit=on
  Logical Operator : Logic  Operator=OR  AllPortsSameDT=off  OutDataTypeStr=boolean
  Logical Operator1 : Logic  Operator=OR  AllPortsSameDT=off  OutDataTypeStr=boolean
  Merge : Merge  Inputs=15
  Subsystem3 : Subsystem
  Sum : Sum  Inputs=|++++++++++++++
  Switch Case : SwitchCase  CaseConditions={1 2 3 4 5 6 7 0 -1 -2 -3 -4 -5 -6 -7}  ShowDefaultCase=off
  tag scope: bS10=global, bS1=global, bS2=global, bS3=global, bS4=global, bS5=global, bS6=global, bS7=global, bS8=global, bS9=global, bVref=global
  wires:
  Constant1/1 -> If Action Subsystem/1(In1)
  Constant2/1 -> If Action Subsystem1/1(In1)
  Constant3/1 -> If Action Subsystem2/1(In1)
  Constant4/1 -> If Action Subsystem3/1(In1)
  Constant5/1 -> If Action Subsystem4/1(In1)
  If Action Subsystem/1(Out1) -> Merge/1
  If Action Subsystem1/1(Out1) -> Merge/2
  If Action Subsystem2/1(Out1) -> Merge/3
  If Action Subsystem3/1(Out1) -> Merge/4
  If Action Subsystem4/1(Out1) -> Merge/5
  Merge/1 -> Demux/1
  Demux/2 -> [bS2]
  Demux/3 -> [bS3]
  Demux/4 -> [bS4]
  Demux/1 -> [bS1]
  Demux/5 -> [bS5]
  Constant6/1 -> If Action Subsystem5/1(In1)
  Constant7/1 -> If Action Subsystem6/1(In1)
  If Action Subsystem6/1(Out1) -> Merge/7
  If Action Subsystem5/1(Out1) -> Merge/6
  Demux/6 -> [bS6]
  Demux/7 -> [bS7]
  Constant8/1 -> If Action Subsystem7/1(In1)
  Constant9/1 -> If Action Subsystem8/1(In1)
  If Action Subsystem8/1(Out1) -> Merge/9
  If Action Subsystem7/1(Out1) -> Merge/8
  Switch Case/1 -> If Action Subsystem/Action
  Switch Case/2 -> If Action Subsystem1/Action
  Switch Case/3 -> If Action Subsystem2/Action
  Switch Case/4 -> If Action Subsystem3/Action
  Switch Case/5 -> If Action Subsystem4/Action
  Switch Case/6 -> If Action Subsystem5/Action
  Switch Case/7 -> If Action Subsystem6/Action
  Switch Case/8 -> If Action Subsystem7/Action
  Switch Case/9 -> If Action Subsystem8/Action
  Constant10/1 -> If Action Subsystem9/1(In1)
  Constant11/1 -> If Action Subsystem10/1(In1)
  Constant12/1 -> If Action Subsystem11/1(In1)
  Constant13/1 -> If Action Subsystem12/1(In1)
  Constant14/1 -> If Action Subsystem13/1(In1)
  If Action Subsystem9/1(Out1) -> Merge/10
  If Action Subsystem10/1(Out1) -> Merge/11
  If Action Subsystem12/1(Out1) -> Merge/13
  If Action Subsystem13/1(Out1) -> Merge/14
  Constant15/1 -> If Action Subsystem14/1(In1)
  Switch Case/11 -> If Action Subsystem10/Action
  Switch Case/12 -> If Action Subsystem11/Action
  Switch Case/13 -> If Action Subsystem12/Action
  Switch Case/14 -> If Action Subsystem13/Action
  Switch Case/15 -> If Action Subsystem14/Action
  Switch Case/10 -> If Action Subsystem9/Action
  If Action Subsystem11/1(Out1) -> Merge/12
  If Action Subsystem14/1(Out1) -> Merge/15
  Demux/8 -> [bS8]
  Subsystem3/1(Out1) -> Sum/1
  Subsystem3/6(Out6) -> Sum/6
  Subsystem3/7(Out7) -> Sum/7
  Subsystem3/10(Out10) -> Sum/10
  Subsystem3/9(Out9) -> Sum/9
  Subsystem3/8(Out8) -> Sum/8
  Subsystem3/5(Out5) -> Sum/5
  Subsystem3/4(Out4) -> Sum/4
  Subsystem3/2(Out2) -> Sum/2
  Subsystem3/3(Out3) -> Sum/3
  Subsystem3/14(Out14) -> Sum/14
  Subsystem3/12(Out12) -> Sum/12
  Subsystem3/13(Out13) -> Sum/13
  Subsystem3/11(Out11) -> Sum/11
  Sum/1 -> [bVref], Switch Case/1
  Demux/9 -> Logical Operator/2
  Logical Operator/1 -> [bS9]
  Logical Operator1/1 -> [bS10]
  Demux/10 -> Logical Operator1/2

== system mytopologybat/Subsystem6/Subsystem1/Subsystem1/If Action Subsystem ==
  In1 : Inport
  Action Port : ActionPort  ActionType=case
  Out1 : Outport
  wires:
  In1/1 -> Out1/1

== system mytopologybat/Subsystem6/Subsystem1/Subsystem1/If Action Subsystem1 ==
  In1 : Inport
  Action Port : ActionPort  ActionType=case
  Out1 : Outport
  wires:
  In1/1 -> Out1/1

== system mytopologybat/Subsystem6/Subsystem1/Subsystem1/If Action Subsystem10 ==
  In1 : Inport
  Action Port : ActionPort  ActionType=case
  Out1 : Outport
  wires:
  In1/1 -> Out1/1

== system mytopologybat/Subsystem6/Subsystem1/Subsystem1/If Action Subsystem11 ==
  In1 : Inport
  Action Port : ActionPort  ActionType=case
  Out1 : Outport
  wires:
  In1/1 -> Out1/1

== system mytopologybat/Subsystem6/Subsystem1/Subsystem1/If Action Subsystem12 ==
  In1 : Inport
  Action Port : ActionPort  ActionType=case
  Out1 : Outport
  wires:
  In1/1 -> Out1/1

== system mytopologybat/Subsystem6/Subsystem1/Subsystem1/If Action Subsystem13 ==
  In1 : Inport
  Action Port : ActionPort  ActionType=case
  Out1 : Outport
  wires:
  In1/1 -> Out1/1

== system mytopologybat/Subsystem6/Subsystem1/Subsystem1/If Action Subsystem14 ==
  In1 : Inport
  Action Port : ActionPort  ActionType=case
  Out1 : Outport
  wires:
  In1/1 -> Out1/1

== system mytopologybat/Subsystem6/Subsystem1/Subsystem1/If Action Subsystem2 ==
  In1 : Inport
  Action Port : ActionPort  ActionType=case
  Out1 : Outport
  wires:
  In1/1 -> Out1/1

== system mytopologybat/Subsystem6/Subsystem1/Subsystem1/If Action Subsystem3 ==
  In1 : Inport
  Action Port : ActionPort  ActionType=case
  Out1 : Outport
  wires:
  In1/1 -> Out1/1

== system mytopologybat/Subsystem6/Subsystem1/Subsystem1/If Action Subsystem4 ==
  In1 : Inport
  Action Port : ActionPort  ActionType=case
  Out1 : Outport
  wires:
  In1/1 -> Out1/1

== system mytopologybat/Subsystem6/Subsystem1/Subsystem1/If Action Subsystem5 ==
  In1 : Inport
  Action Port : ActionPort  ActionType=case
  Out1 : Outport
  wires:
  In1/1 -> Out1/1

== system mytopologybat/Subsystem6/Subsystem1/Subsystem1/If Action Subsystem6 ==
  In1 : Inport
  Action Port : ActionPort  ActionType=case
  Out1 : Outport
  wires:
  In1/1 -> Out1/1

== system mytopologybat/Subsystem6/Subsystem1/Subsystem1/If Action Subsystem7 ==
  In1 : Inport
  Action Port : ActionPort  ActionType=case
  Out1 : Outport
  wires:
  In1/1 -> Out1/1

== system mytopologybat/Subsystem6/Subsystem1/Subsystem1/If Action Subsystem8 ==
  In1 : Inport
  Action Port : ActionPort  ActionType=case
  Out1 : Outport
  wires:
  In1/1 -> Out1/1

== system mytopologybat/Subsystem6/Subsystem1/Subsystem1/If Action Subsystem9 ==
  In1 : Inport
  Action Port : ActionPort  ActionType=case
  Out1 : Outport
  wires:
  In1/1 -> Out1/1

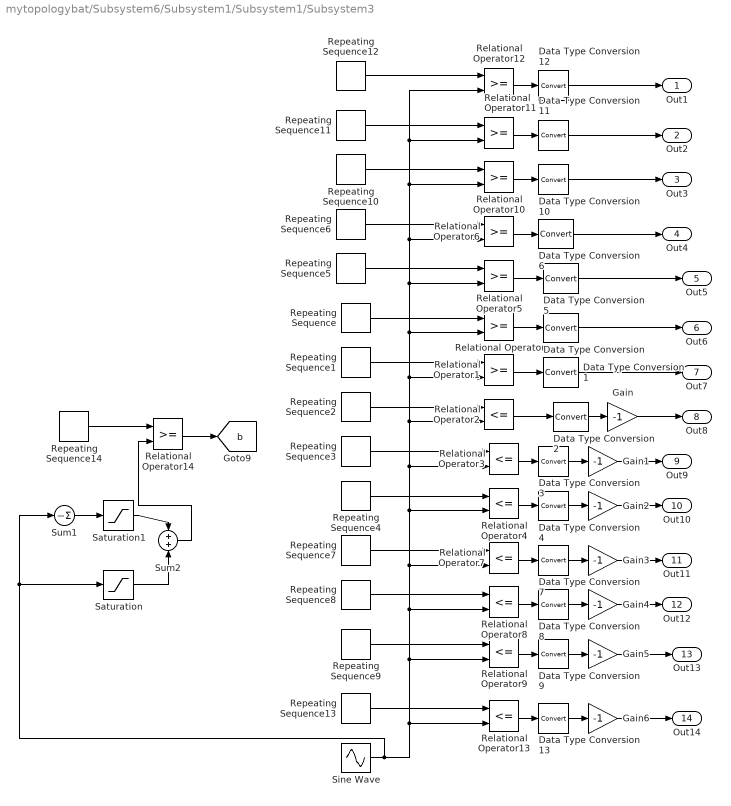
== system mytopologybat/Subsystem6/Subsystem1/Subsystem1/Subsystem3 ==
  Data Type Conversion{,1..13} (14 alike) : DataTypeConversion
  Gain{,1..6} (7 alike) : Gain  Gain=-1
  Relational Operator{,1,5..6,10..12,14} (8 alike) : RelationalOperator  OutDataTypeStr=boolean
  Relational Operator{2..4,7..9,13} (7 alike) : RelationalOperator  Operator=<=  OutDataTypeStr=boolean
  Repeating Sequence : simulink/Sources/Repeating Sequence  rep_seq_t="[0 (1/fc)/2  (1/fc)]"  rep_seq_y=[1 2 1]
  Repeating Sequence1 : simulink/Sources/Repeating Sequence  rep_seq_t="[0 (1/fc)/2  (1/fc)]"  rep_seq_y=[0 1 0]
  Repeating Sequence10 : simulink/Sources/Repeating Sequence  rep_seq_t="[0 (1/fc)/2  (1/fc)]"  rep_seq_y=[4 5 4]
  Repeating Sequence11 : simulink/Sources/Repeating Sequence  rep_seq_t="[0 (1/fc)/2  (1/fc)]"  rep_seq_y=[5 6 5]
  Repeating Sequence12 : simulink/Sources/Repeating Sequence  rep_seq_t="[0 (1/fc)/2  (1/fc)]"  rep_seq_y=[6 7 6]
  Repeating Sequence13 : simulink/Sources/Repeating Sequence  rep_seq_t="[0 (1/fc)/2  (1/fc)]"  rep_seq_y=[-7 -6 -7]
  Repeating Sequence14 : simulink/Sources/Repeating Sequence  rep_seq_t="[0 (1/fc)/2  (1/fc)]"  rep_seq_y=[0 1 0]
  Repeating Sequence2 : simulink/Sources/Repeating Sequence  rep_seq_t="[0 (1/fc)/2  (1/fc)]"  rep_seq_y=[-1 0 -1]
  Repeating Sequence3 : simulink/Sources/Repeating Sequence  rep_seq_t="[0 (1/fc)/2  (1/fc)]"  rep_seq_y=[-2 -1 -2]
  Repeating Sequence4 : simulink/Sources/Repeating Sequence  rep_seq_t="[0 (1/fc)/2  (1/fc)]"  rep_seq_y=[-3 -2 -3]
  Repeating Sequence5 : simulink/Sources/Repeating Sequence  rep_seq_t="[0 (1/fc)/2  (1/fc)]"  rep_seq_y=[2 3 2]
  Repeating Sequence6 : simulink/Sources/Repeating Sequence  rep_seq_t="[0 (1/fc)/2  (1/fc)]"  rep_seq_y=[3 4 3]
  Repeating Sequence7 : simulink/Sources/Repeating Sequence  rep_seq_t="[0 (1/fc)/2  (1/fc)]"  rep_seq_y=[-4 -3 -4]
  Repeating Sequence8 : simulink/Sources/Repeating Sequence  rep_seq_t="[0 (1/fc)/2  (1/fc)]"  rep_seq_y=[-5 -4 -5]
  Repeating Sequence9 : simulink/Sources/Repeating Sequence  rep_seq_t="[0 (1/fc)/2  (1/fc)]"  rep_seq_y=[-6 -5 -6]
  Saturation : Saturate  UpperLimit=10  LowerLimit=0
  Saturation1 : Saturate  UpperLimit=10  LowerLimit=0
  Sine Wave : Sin  Amplitude=7*m  Frequency=2*pi*50  Phase=2*pi/3  SampleTime=0
  Sum1 : Sum  Inputs=-
  Sum2 : Sum
  Out1 : Outport
  Out2 : Outport  Port=2
  Out3 : Outport  Port=3
  Out4 : Outport  Port=4
  Out5 : Outport  Port=5
  Out6 : Outport  Port=6
  Out7 : Outport  Port=7
  Out8 : Outport  Port=8
  Out9 : Outport  Port=9
  Out10 : Outport  Port=10
  Out11 : Outport  Port=11
  Out12 : Outport  Port=12
  Out13 : Outport  Port=13
  Out14 : Outport  Port=14
  tag scope: b=global
  wires:
  Relational Operator/1 -> Data Type Conversion/1
  Relational Operator1/1 -> Data Type Conversion1/1
  Repeating Sequence/1 -> Relational Operator/1
  Repeating Sequence1/1 -> Relational Operator1/1
  Repeating Sequence2/1 -> Relational Operator2/1
  Repeating Sequence3/1 -> Relational Operator3/1
  Relational Operator2/1 -> Data Type Conversion2/1
  Relational Operator3/1 -> Data Type Conversion3/1
  Data Type Conversion2/1 -> Gain/1
  Data Type Conversion3/1 -> Gain1/1
  Repeating Sequence4/1 -> Relational Operator4/1
  Relational Operator4/1 -> Data Type Conversion4/1
  Data Type Conversion4/1 -> Gain2/1
  Relational Operator5/1 -> Data Type Conversion5/1
  Repeating Sequence5/1 -> Relational Operator5/1
  Relational Operator6/1 -> Data Type Conversion6/1
  Repeating Sequence6/1 -> Relational Operator6/1
  Repeating Sequence7/1 -> Relational Operator7/1
  Relational Operator7/1 -> Data Type Conversion7/1
  Data Type Conversion7/1 -> Gain3/1
  Repeating Sequence8/1 -> Relational Operator8/1
  Relational Operator8/1 -> Data Type Conversion8/1
  Data Type Conversion8/1 -> Gain4/1
  Repeating Sequence9/1 -> Relational Operator9/1
  Relational Operator9/1 -> Data Type Conversion9/1
  Data Type Conversion9/1 -> Gain5/1
  Repeating Sequence10/1 -> Relational Operator10/1
  Relational Operator10/1 -> Data Type Conversion10/1
  Repeating Sequence11/1 -> Relational Operator11/1
  Relational Operator11/1 -> Data Type Conversion11/1
  Relational Operator12/1 -> Data Type Conversion12/1
  Repeating Sequence12/1 -> Relational Operator12/1
  Repeating Sequence13/1 -> Relational Operator13/1
  Relational Operator13/1 -> Data Type Conversion13/1
  Data Type Conversion13/1 -> Gain6/1
  Data Type Conversion12/1 -> Out1/1
  Data Type Conversion11/1 -> Out2/1
  Data Type Conversion10/1 -> Out3/1
  Data Type Conversion6/1 -> Out4/1
  Data Type Conversion5/1 -> Out5/1
  Data Type Conversion/1 -> Out6/1
  Data Type Conversion1/1 -> Out7/1
  Gain/1 -> Out8/1
  Gain1/1 -> Out9/1
  Gain2/1 -> Out10/1
  Gain3/1 -> Out11/1
  Gain4/1 -> Out12/1
  Gain5/1 -> Out13/1
  Gain6/1 -> Out14/1
  Relational Operator14/1 -> [b]
  Sum2/1 -> Relational Operator14/2
  Repeating Sequence14/1 -> Relational Operator14/1
  Saturation/1 -> Sum2/2
  Saturation1/1 -> Sum2/1
  Sum1/1 -> Saturation1/1
  Sine Wave/1 -> Relational Operator13/2, Relational Operator9/2, Relational Operator8/2, Relational Operator7/2, Relational Operator4/2, Relational Operator3/2, Relational Operator2/2, Relational Operator1/2, Relational Operator/2, Relational Operator5/2, Relational Operator6/2, Relational Operator10/2, Relational Operator11/2, Relational Operator12/2, Saturation/1, Sum1/1

== system mytopologybat/Subsystem6/Subsystem2/Subsystem/If Action Subsystem ==
  In1 : Inport
  Action Port : ActionPort  ActionType=case
  Out1 : Outport
  wires:
  In1/1 -> Out1/1

== system mytopologybat/Subsystem6/Subsystem2/Subsystem/If Action Subsystem1 ==
  In1 : Inport
  Action Port : ActionPort  ActionType=case
  Out1 : Outport
  wires:
  In1/1 -> Out1/1

== system mytopologybat/Subsystem6/Subsystem2/Subsystem/If Action Subsystem10 ==
  In1 : Inport
  Action Port : ActionPort  ActionType=case
  Out1 : Outport
  wires:
  In1/1 -> Out1/1

== system mytopologybat/Subsystem6/Subsystem2/Subsystem/If Action Subsystem11 ==
  In1 : Inport
  Action Port : ActionPort  ActionType=case
  Out1 : Outport
  wires:
  In1/1 -> Out1/1

== system mytopologybat/Subsystem6/Subsystem2/Subsystem/If Action Subsystem12 ==
  In1 : Inport
  Action Port : ActionPort  ActionType=case
  Out1 : Outport
  wires:
  In1/1 -> Out1/1

== system mytopologybat/Subsystem6/Subsystem2/Subsystem/If Action Subsystem13 ==
  In1 : Inport
  Action Port : ActionPort  ActionType=case
  Out1 : Outport
  wires:
  In1/1 -> Out1/1

== system mytopologybat/Subsystem6/Subsystem2/Subsystem/If Action Subsystem14 ==
  In1 : Inport
  Action Port : ActionPort  ActionType=case
  Out1 : Outport
  wires:
  In1/1 -> Out1/1

== system mytopologybat/Subsystem6/Subsystem2/Subsystem/If Action Subsystem2 ==
  In1 : Inport
  Action Port : ActionPort  ActionType=case
  Out1 : Outport
  wires:
  In1/1 -> Out1/1

== system mytopologybat/Subsystem6/Subsystem2/Subsystem/If Action Subsystem3 ==
  In1 : Inport
  Action Port : ActionPort  ActionType=case
  Out1 : Outport
  wires:
  In1/1 -> Out1/1

== system mytopologybat/Subsystem6/Subsystem2/Subsystem/If Action Subsystem4 ==
  In1 : Inport
  Action Port : ActionPort  ActionType=case
  Out1 : Outport
  wires:
  In1/1 -> Out1/1

== system mytopologybat/Subsystem6/Subsystem2/Subsystem/If Action Subsystem5 ==
  In1 : Inport
  Action Port : ActionPort  ActionType=case
  Out1 : Outport
  wires:
  In1/1 -> Out1/1

== system mytopologybat/Subsystem6/Subsystem2/Subsystem/If Action Subsystem6 ==
  In1 : Inport
  Action Port : ActionPort  ActionType=case
  Out1 : Outport
  wires:
  In1/1 -> Out1/1

== system mytopologybat/Subsystem6/Subsystem2/Subsystem/If Action Subsystem7 ==
  In1 : Inport
  Action Port : ActionPort  ActionType=case
  Out1 : Outport
  wires:
  In1/1 -> Out1/1

== system mytopologybat/Subsystem6/Subsystem2/Subsystem/If Action Subsystem8 ==
  In1 : Inport
  Action Port : ActionPort  ActionType=case
  Out1 : Outport
  wires:
  In1/1 -> Out1/1

== system mytopologybat/Subsystem6/Subsystem2/Subsystem/If Action Subsystem9 ==
  In1 : Inport
  Action Port : ActionPort  ActionType=case
  Out1 : Outport
  wires:
  In1/1 -> Out1/1
